simulink model "snap_f_12i_2kc"  (R2021a)
settings: Solver=VariableStepDiscrete  StartTime=0.0  StopTime=10.0  RelTol=1e-3
libraries: xbsIndex_r4 x2585, xps_library x8, casper_library_misc x8, casper_library_sources x4, casper_library_delays x2, casper_library_reorder x1, casper_library_communications x1
(part 1 of 32)
settings Model: ModifiedComment=kocz -- Fri Jun 12 15:44:21 2020 -- Version 1.371  Creator=mdexter  LastModifiedBy=jackh
settings Model: ModifiedHistory=|
  | kocz -- Fri Jun 12 15:36:18 2020 -- Version 1.370
  | 
  | Updated initial yellow blocks.
  | 
  | kocz -- Fri Jun 12 15:28:41 2020 -- Version 1.369
  | 
  | Started updating to 2018a. Restarting due to finding casper library bug.
  | 
  | jackh -- Sun Oct 27 09:17:26 2019 -- Version 1.368
  | compiled
  | 
  | jackh -- Sun Oct 27 07:24:12 2019 -- Version 1.367
  | remove registering of reorder outputs
  | 
  | jackh -- Sun Oct 27 07:22:37 2019 -- Version 1.366
  | change input snapshot to snap only one of 3 inputs
  | 
  | jackh -- Sun Oct 27 03:59:18 2019 -- Version 1.365
  | remove some superfluous registers to improve timing.
  | Reduce snapshot in input block from 1k samples to 512
  | 
  | jackh -- Sun Oct 27 01:46:50 2019 -- Version 1.364
  | Fix FFT shift bitwidth bug
  | 
  | FFT core was expecting a 16-bit shift, but only a 12bit value was sliced from the control register
  | 
  | jackh -- Fri Aug 30 09:22:01 2019 -- Version 1.363
  | compiled
  | 
  | jackh -- Thu Aug 29 17:13:27 2019 -- Version 1.362
  | change delay shift reg to 3 bit addr
  | 
  | jackh -- Thu Aug 29 11:33:13 2019 -- Version 1.361
  | corr fixes
  | 
  | jackh -- Thu Aug 29 11:09:21 2019 -- Version 1.360
  | latency fix in eqtvg
  | 
  | jackh -- Thu Aug 29 10:02:04 2019 -- Version 1.359
  | compiled
  | 
  | jackh -- Wed Aug 28 15:31:00 2019 -- Version 1.358
  | bump to version 1.3
  | 
  | jackh -- Wed Aug 28 15:26:18 2019 -- Version 1.357
  | change quantization to saturate.
  | Change coefficients to 16_5 (was 16_6)
  | 
  | jackh -- Wed Aug 28 14:17:28 2019 -- Version 1.356
  | remove debugging snapshots hidden in corr vaccs
  | 
  | jackh -- Fri Aug 23 15:01:55 2019 -- Version 1.355
  | compiled
  | 
  | jackh -- Fri Aug 23 10:43:05 2019 -- Version 1.354
  | add snapshot in input block
  | 
  | jackh -- Thu Aug 22 17:13:50 2019 -- Version 1.353
  | fix to eqtvg ram depths
  | 
  | jackh -- Thu Aug 22 15:23:14 2019 -- Version 1.352
  | bump version to 1.2
  | 
  | jackh -- Thu Aug 22 15:22:39 2019 -- Version 1.351
  | Force pairs of pols to have same random number generator to save resources
  | 
  | jackh -- Thu Aug 22 15:19:21 2019 -- Version 1.350
  | rotator channel index counter fixes
  | 
  | eq tvg split bram into 3 (so we can have 6 channels, not 8)
  | 
  | jackh -- Thu Aug 22 12:01:44 2019 -- Version 1.349
  | 
  | 
  | jackh -- Thu Aug 22 12:01:21 2019 -- Version 1.348
  | Changes to rotator precision
  | 
  | jackh -- Tue Aug 20 19:46:09 2019 -- Version 1.347
  | compiled
  | 
  | jackh -- Tue Aug 20 16:55:38 2019 -- Version 1.346
  | increase minimum walsh period to 2**18 fpga clocks (was 2**13)
  | 
  | jackh -- Tue Aug 20 16:40:34 2019 -- Version 1.345
  | 
  | 
  | jackh -- Tue Aug 20 16:15:18 2019 -- Version 1.344
  | bump version to 1.1
  | 
  | jackh -- Tue Aug 20 16:14:49 2019 -- Version 1.343
  | add global enables to phase switch mod/demod to make software easier
  | 
  | jackh -- Mon Aug 19 17:54:23 2019 -- Version 1.342
  | compiled
  | 
  | jackh -- Thu Aug 01 11:53:22 2019 -- Version 1.341
  | make programmable sync delay tolerate delay=0
  | 
  | jackh -- Wed Jul 31 13:49:54 2019 -- Version 1.340
  | comment out corr->rms
  | 
  | jackh -- Mon Jul 29 17:05:34 2019 -- Version 1.339
  | delete corr rms block (not currently enough ram)
  | 
  | jackh -- Mon Jul 29 17:03:29 2019 -- Version 1.338
  | Add version block
  | 
  | jackh -- Mon Jul 29 16:58:22 2019 -- Version 1.337
  | make sync in have a programmable delay
  | Solves 2 problems:
  | 
  | 1) Can start integrations at arbitrary times (good for LST alignment)
  | 2) Can start a 16 second integration chunk on an arbitrary time boundary (needed to avoid the downstream correlator having 16 second start / stop granularity)
  | 
  | jackh -- Mon Jul 29 16:50:03 2019 -- Version 1.336
  | update phasor to 24-bits
  | 
  | jackh -- Sat May 11 17:48:41 2019 -- Version 1.335
  | 
  | 
  | jackh -- Sat May 11 17:46:07 2019 -- Version 1.334
  | 
  | 
  | jackh -- Sat May 11 17:45:44 2019 -- Version 1.333
  | 
  | 
  | jackh -- Sat May 11 17:40:04 2019 -- Version 1.332
  | 
  | 
  | jackh -- Sat May 11 17:36:59 2019 -- Version 1.331
  | add vacc for autocorrs @ 16 bit resolution
  | 
  | deepthi -- Sun Oct 28 15:16:19 2018 -- Version 1.330
  | 
  | 
  | deepthi -- Sat Oct 27 18:45:54 2018 -- Version 1.329
  | 
  | packetizer: Added an 'and' block that holds new_packet signal in high until the first sync.
  | 
  | deepthi -- Sat Oct 27 17:33:32 2018 -- Version 1.328
  | 
  | 1. Change edge_detect location in sync block
  | 
  | deepthi -- Sat Oct 20 22:13:43 2018 -- Version 1.327
  | 
  | 1. Add edge detect to software reg and gpio input in sync block.
  | 
  | 2. Add new corr block with max hold functionality.
  | 
  | jackh -- Tue Oct 09 20:34:13 2018 -- Version 1.326
  | recompile with pmbus_alert register
  | 
  | jackh -- Thu Jul 12 10:55:28 2018 -- Version 1.325
  | 
  | 
  | jackh -- Wed Jul 11 17:20:51 2018 -- Version 1.324
  | syntax
  | 
  | jackh -- Wed Jul 11 17:16:24 2018 -- Version 1.323
  | increase resolution of phase rotator bram.
  | 
  | jackh -- Wed Jul 11 17:10:41 2018 -- Version 1.322
  | 
  | 
  | jackh -- Tue Jul 10 16:08:30 2018 -- Version 1.321
  | scramble rotator channel multiplers to match PFB output order (hopefully)
  | 
  | jackh -- Tue Jul 10 15:51:56 2018 -- Version 1.320
  | 
  | 
  | jackh -- Tue Jul 10 13:37:24 2018 -- Version 1.319
  | fix off-by-one in slicing of mcnt counter, which was having the effect of duplicating mcnts in headers
  | 
  | jackh -- Sat Jul 07 14:17:05 2018 -- Version 1.318
  | compiled
  | 
  | jackh -- Fri Jul 06 10:33:47 2018 -- Version 1.317
  | fix bitbashing to rotator phase addresses
  | 
  | jackh -- Fri Jul 06 10:17:15 2018 -- Version 1.316
  | Add mux to enable / disable rotator
  | 
  | jackh -- Thu Jul 05 17:21:10 2018 -- Version 1.315
  | make some delays behavioural
  | 
  | jackh -- Thu Jul 05 14:48:28 2018 -- Version 1.314
  | 
  | 
  | jackh -- Thu Jul 05 14:46:13 2018 -- Version 1.313
  | 
  | 
  | jackh -- Thu Jul 05 14:43:36 2018 -- Version 1.312
  | 
  | 
  | jackh -- Thu Jul 05 14:40:00 2018 -- Version 1.311
  | 
  | 
  | jackh -- Thu Jul 05 14:36:19 2018 -- Version 1.310
  | 
  | 
  | jackh -- Thu Jul 05 14:26:16 2018 -- Version 1.309
  | integrate rotator into pipeline
  | 
  | jackh -- Thu Jul 05 14:20:20 2018 -- Version 1.308
  | 
  | create phase-rotation block
  | 
  | deepthi -- Thu Jun 07 09:24:03 2018 -- Version 1.307
  | 
  | Replaced the corr block.
  | 
  | deepthi -- Wed Jun 06 12:07:26 2018 -- Version 1.306
  | 
  | 
  | deepthi -- Tue Jun 05 17:46:17 2018 -- Version 1.305
  | 
  | Replaced the corr block with the tested version
  | 
  | deepthi -- Sat May 12 19:11:02 2018 -- Version 1.304
  | 
  | Changed time counter to increment between even/odd banks
  | 
  | deepthi -- Sat May 12 19:06:34 2018 -- Version 1.303
  | 
  | changed timing of eof, valid, data and headers
  | 
  | deepthi -- Mon May 07 23:03:07 2018 -- Version 1.302
  | 
  | 
  | deepthi -- Mon May 07 00:31:44 2018 -- Version 1.301
  | 
  | 
  | deepthi -- Fri May 04 20:13:43 2018 -- Version 1.300
  | 
  | Reduced width sliced from time_ctr
  | 
  | deepthi -- Fri May 04 19:47:57 2018 -- Version 1.299
  | 
  | Added delay to header and ip signals to account for pulse_ext on valid.
  | 
  | deepthi -- Fri May 04 19:23:23 2018 -- Version 1.298
  | 
  | 
  | deepthi -- Thu May 03 16:58:39 2018 -- Version 1.297
  | 
  | 1. Added delays to eof and dest_ip  to account for pulse_ext in valid.
  | 
  | 2. Changed eth_sw expected packet length to include header.
  | 
  | jackh -- Tue May 01 20:38:09 2018 -- Version 1.296
  | compiled
  | 
  | jackh -- Tue May 01 17:49:38 2018 -- Version 1.295
  | Fix to packetizer valid generation, to take into account the 3 (one per antenna) blocks of valid data in each stream of 512 channels
  | 
  | jackh -- Tue May 01 16:49:02 2018 -- Version 1.294
  | make channel selection bram 32-bits wide.
  | 
  | Remove GPU-packing mux / swreg
  | 
  | jackh -- Tue May 01 14:24:16 2018 -- Version 1.293
  | 
  | 
  | jackh -- Tue May 01 14:20:01 2018 -- Version 1.292
  | update chan reorderer
  | 
  | jackh -- Tue May 01 11:43:41 2018 -- Version 1.291
  | compiled
  | 
  | jackh -- Tue May 01 09:44:03 2018 -- Version 1.290
  | 
  | 
  | jackh -- Tue May 01 09:43:34 2018 -- Version 1.289
  | use bram for eq fft descramble map
  | 
  | jackh -- Tue May 01 09:40:26 2018 -- Version 1.288
  | change architecture of corr block -- now stores desired antennas in bram, rather than using a delay tree
  | 
  | jackh -- Mon Apr 30 20:21:35 2018 -- Version 1.287
  | 
  | 
  | jackh -- Mon Apr 30 20:18:20 2018 -- Version 1.286
  | 
  | 
  | jackh -- Mon Apr 30 20:15:51 2018 -- Version 1.285
  | compensate for FFT scrambling in EQ block. Descramble FFT post-requantization in this block
  | 
  | jackh -- Mon Apr 30 19:27:42 2018 -- Version 1.284
  | plausibility pass on corr block
  | 
  | jackh -- Mon Apr 30 12:16:47 2018 -- Version 1.283
  | 
  | 
  | jackh -- Mon Apr 30 12:14:25 2018 -- Version 1.282
  | store chan_reorder reorder map in bram
  | 
  | jackh -- Mon Apr 30 12:05:02 2018 -- Version 1.281
  | remove per-antenna histograms -- now get one histogram with multiplexed input
  | 
  | jackh -- Sun Apr 29 15:50:16 2018 -- Version 1.280
  | 
  | 
  | jackh -- Sun Apr 29 15:37:38 2018 -- Version 1.279
  | 
  | 
  | jackh -- Sun Apr 29 15:27:38 2018 -- Version 1.278
  | First pass packetizer. Regenerate pfb with parameter for serial block inputs
  | 
  | jackh -- Sat Mar 03 12:52:57 2018 -- Version 1.277
  | 
  | 
  | jackh -- Sun Feb 25 12:27:48 2018 -- Version 1.276
  | add pre-pfb reorder
  | 
  | jackh -- Sat Feb 24 13:39:06 2018 -- Version 1.275
  | 
  | jackh -- Sat Feb 24 13:38:40 2018 -- Version 1.274
  | update pfb to 16 inputs
  | 
  | jackh -- Fri Feb 23 18:44:26 2018 -- Version 1.273
  | 
  | 
  | jackh -- Fri Feb 23 18:38:20 2018 -- Version 1.272
  | 
  | 
  | jackh -- Fri Feb 23 17:01:30 2018 -- Version 1.271
  | make fft 8 parallel input
  | 
  | jackh -- Sat Feb 10 13:53:12 2018 -- Version 1.270
  | 
  | 
  | jackh -- Sat Feb 10 13:50:10 2018 -- Version 1.269
  | 
  | 
  | jackh -- Sat Feb 10 13:48:56 2018 -- Version 1.268
  | remove fft preshift
  | 
  | jackh -- Sat Feb 10 13:47:39 2018 -- Version 1.267
  | 
  | 
  | jackh -- Sat Feb 10 13:44:29 2018 -- Version 1.266
  | 
  | 
  | jackh -- Sat Feb 10 13:43:22 2018 -- Version 1.265
  | make delayer dual-pol
  | 
  | jackh -- Sat Feb 10 13:40:59 2018 -- Version 1.264
  | first pass new packet format with no time-based corner turn
  | 
  | jackh -- Fri Feb 09 17:29:05 2018 -- Version 1.263
  | 
  | 
  | jackh -- Fri Feb 09 15:23:03 2018 -- Version 1.262
  | first pass turning everything to 8192 channels
  | 
  | Changed the ants addr to be driven by the same signal that drives chans, ips (used to be driven by ant_tracker).
  | 
  | Removed nants software register that was previously thought to control time stamps (but didn't really)
  | 
  | deepthi -- Wed Jan 31 18:20:45 2018 -- Version 1.261
  | 
  | deepthi -- Mon Jan 29 17:20:36 2018 -- Version 1.260
  | 
  | 
  | deepthi -- Mon Jan 29 17:18:54 2018 -- Version 1.259
  | 
  | 
  | deepthi -- Mon Jan 29 17:18:33 2018 -- Version 1.258
  | 
  | 
  | deepthi -- Mon Jan 29 16:51:19 2018 -- Version 1.257
  | 
  | 
  | deepthi -- Mon Jan 29 16:46:46 2018 -- Version 1.256
  | 
  | 
  | deepthi -- Mon Jan 29 16:37:32 2018 -- Version 1.255
  | 
  | 
  | deepthi -- Mon Jan 29 16:11:03 2018 -- Version 1.254
  | 
  | 
  | deepthi -- Mon Jan 29 15:55:33 2018 -- Version 1.253
  | 
  | 
  | jackh -- Fri Nov 17 19:04:05 2017 -- Version 1.252
  | compiled
  | 
  | jackh -- Wed Nov 15 11:31:03 2017 -- Version 1.251
  | go to 3 corr blocks
  | 
  | jackh -- Tue Nov 14 16:10:40 2017 -- Version 1.250
  | 
  | 
  | jackh -- Tue Nov 14 15:28:37 2017 -- Version 1.249
  | reduce bram use in histogram shared brams
  | 
  | jackh -- Mon Nov 13 18:55:18 2017 -- Version 1.248
  | fix bug in histogram shared bram addr width
  | 
  | jackh -- Fri Nov 10 17:05:56 2017 -- Version 1.247
  | add 4 independent corr subsystems. Add EQ clipping counters
  | 
  | jackh -- Fri Nov 10 14:21:14 2017 -- Version 1.246
  | 
  | 
  | jackh -- Fri Nov 10 14:19:27 2017 -- Version 1.245
  | 
  | 
  | jackh -- Fri Nov 10 11:40:47 2017 -- Version 1.244
  | update to histograms v2
  | 
  | jackh -- Tue Nov 07 22:23:59 2017 -- Version 1.243
  | compiled -- passes eqtvg
  | 
  | jackh -- Tue Nov 07 20:41:00 2017 -- Version 1.242
  | 
  | 
  | jackh -- Tue Nov 07 20:39:30 2017 -- Version 1.241
  | packet header generation fixes
  | 
  | jackh -- Tue Nov 07 17:19:53 2017 -- Version 1.240
  | 
  | 
  | jackh -- Tue Nov 07 17:14:47 2017 -- Version 1.239
  | 
  | 
  | jackh -- Tue Nov 07 17:08:29 2017 -- Version 1.238
  | remove some chan_reorder debug snapshots
  | 
  | jackh -- Tue Nov 07 17:06:39 2017 -- Version 1.237
  | update ps GPIO pins
  | 
  | **** Change packetizer header blocks to can have a separate antenna / ip / chan for each packet. This is for the nants > 3 simulation modes. This will break previous versions of software *****
  | 
  | jackh -- Mon Nov 06 22:06:03 2017 -- Version 1.236
  | add comment to corr_acc_len
  | 
  | Compiled -- passes EQTVG test!
  | 
  | jackh -- Mon Nov 06 15:24:31 2017 -- Version 1.235
  | add OR block in mrst generator so that counter is enabled if/when an arm signal comes
  | 
  | jackh -- Sun Nov 05 21:39:25 2017 -- Version 1.234
  | comment on sync period
  | 
  | jackh -- Sun Nov 05 17:39:01 2017 -- Version 1.233
  | fix bitbasher in 32-spectra corner turn
  | 
  | jackh -- Sun Nov 05 17:05:17 2017 -- Version 1.232
  | aesthetic
  | 
  | jackh -- Sun Nov 05 17:02:53 2017 -- Version 1.231
  | changes to comments
  | 
  | jackh -- Sun Nov 05 17:01:27 2017 -- Version 1.230
  | make acc_len it's own register so we can acc to 2**32
  | 
  | jackh -- Sun Nov 05 16:58:57 2017 -- Version 1.229
  | 
  | 
  | jackh -- Sun Nov 05 16:56:52 2017 -- Version 1.228
  | add internal correlator
  | 
  | jackh -- Sun Nov 05 16:24:21 2017 -- Version 1.227
  | compiled.
  | 
  | jackh -- Sun Nov 05 15:19:13 2017 -- Version 1.226
  | latency tweak to data line in packetizer
  | 
  | jackh -- Sat Nov 04 20:21:54 2017 -- Version 1.225
  | change ethernet debug counters to 32 bits
  | 
  | jackh -- Sat Nov 04 20:05:10 2017 -- Version 1.224
  | make chan reorder map bram 32 bits to aid with software
  | 
  | jackh -- Sat Nov 04 19:51:25 2017 -- Version 1.223
  | change header brams to be 32-bit wide for all values.
  | This makes it easier to deal with the software, which can only write 32-bit bounded words.
  | 
  | jackh -- Sat Nov 04 14:23:39 2017 -- Version 1.222
  | replace big distributed ram in 16-spectra corner turn
  | with simple bit basher manipulation. The distributed ram tool a ridiculous amount of time to synthesize. Hopefully this will be faster.
  | 
  | jackh -- Fri Nov 03 16:25:40 2017 -- Version 1.221
  | 
  | 
  | jackh -- Fri Nov 03 16:17:13 2017 -- Version 1.220
  | update casper blocks on phase switch subsys
  | 
  | jackh -- Fri Nov 03 16:14:34 2017 -- Version 1.219
  | 
  | 
  | jackh -- Fri Nov 03 13:09:23 2017 -- Version 1.218
  | add phase switching and i2c control
  | 
  | jackh -- Fri Nov 03 12:43:29 2017 -- Version 1.217
  | 
  | add i2C controllers
  | 
  | jackh -- Mon Oct 23 16:15:14 2017 -- Version 1.216
  | Add back in Deepthi's fix from f3b63dae07d62
  | 
  | jackh -- Mon Oct 23 16:04:59 2017 -- Version 1.215
  | 
  | 
  | jackh -- Mon Oct 23 14:44:02 2017 -- Version 1.214
  | compiled. Still minor timing errors in the histograms
  | 
  | jackh -- Mon Oct 23 10:40:37 2017 -- Version 1.213
  | change EQ coeffs to one-per channel. Make format 16_6 (was 18_7)
  | 
  | jackh -- Mon Oct 09 15:00:17 2017 -- Version 1.212
  | 
  | halve number of brams in histogram readout
  | 
  | jackh -- Wed Sep 13 11:46:17 2017 -- Version 1.211
  | use built-in tge status regs
  | 
  | jackh -- Tue Sep 12 21:14:25 2017 -- Version 1.210
  | 
  | 
  | jackh -- Tue Sep 12 21:10:57 2017 -- Version 1.209
  | update_casper_blocks(bdroot)
  | 
  | jackh -- Tue Sep 12 21:02:11 2017 -- Version 1.208
  | add histogram to adc stats
  | 
  | jackh -- Fri Jul 14 11:30:38 2017 -- Version 1.207
  | set map = reord_map in chan_reorder blocks which use matlab scripts to generate their reorders.
  | 
  | jackh -- Thu Jul 13 17:48:05 2017 -- Version 1.206
  | change sync period to a 32-bit sw reg (was hardcoded 9! * 1024)
  | 
  | deepthi -- Thu Jul 13 13:07:36 2017 -- Version 1.205
  | 
  | 
  | deepthi -- Thu Jul 13 12:10:35 2017 -- Version 1.204
  | 
  | 
  | deepthi -- Wed Jul 12 16:52:46 2017 -- Version 1.203
  | 
  | 
  | deepthi -- Wed Jul 12 15:57:48 2017 -- Version 1.202
  | 
  | 
  | deepthi -- Tue Jul 11 19:00:41 2017 -- Version 1.201
  | 
  | 
  | deepthi -- Tue Jul 11 18:54:05 2017 -- Version 1.200
  | 
  | 
  | deepthi -- Tue Jul 11 18:52:32 2017 -- Version 1.199
  | 
  | 
  | deepthi -- Mon Jul 10 16:18:51 2017 -- Version 1.198
  | 
  | 
  | deepthi -- Sun Jul 09 18:15:02 2017 -- Version 1.197
  | 
  | 
  | deepthi -- Thu Jul 06 13:54:16 2017 -- Version 1.196
  | 
  | 
  | jackh -- Mon Jul 03 11:01:40 2017 -- Version 1.195
  | 
  | 
  | jackh -- Fri Jun 30 13:59:17 2017 -- Version 1.194
  | enable CPU tx/rx buffer on tge core. Needed for microblaze.
  | 
  | jackh -- Mon Jun 26 11:33:24 2017 -- Version 1.193
  | 
  | 
  | jackh -- Thu Jun 22 14:37:16 2017 -- Version 1.192
  | add history prompting
settings SolverCC: AlgebraicLoopSolver=TrustRegion
settings DataIOCC: LimitDataPoints=on  SaveFormat=Array  SignalLoggingSaveFormat=ModelDataLogs  ReturnWorkspaceOutputs=off
settings OptimizationCC: DefaultParameterBehavior=Inlined  ExpressionDepthLimit=2147483647  LifeSpan=inf
settings DebuggingCC: UnderspecifiedInitializationDetection=Classic  MergeDetectMultiDrivingBlocksExec=none  SolverPrmCheckMsg=warning  FcnCallInpInsideContextMsg=warning  AllowSymbolicDim=off  StateNameClashWarn=warning  SFUnexpectedBacktrackingDiag=warning  SFNoUnconditionalDefaultTransitionDiag=warning  SFExecutionAtInitializationDiag=none  SFMachineParentedDataDiag=warning  ArithmeticOperatorsInVariantConditions=warning
settings HardwareCC: ProdBitPerPointer=32  ProdBitPerSizeT=32  ProdBitPerPtrDiffT=32  ProdLargestAtomicFloat=None  ProdIntDivRoundTo=Undefined  ProdEndianess=Unspecified  ProdWordSize=32  ProdHWDeviceType=32-bit Generic
settings ModelReferenceCC: PropagateSignalLabelsOutOfModel=off
settings SFSimCC: SimUseLocalCustomCode=off  CustomCodeUndefinedFunction=UseInterfaceOnly
settings RTWCC: RTWUseLocalCustomCode=off
settings CodeAppCC: StateflowObjectComments=on
settings GRTTargetCC: TargetLangStandard=C89/C90 (ANSI)  CombineOutputUpdateFcns=off  GRTInterface=on
settings ConfigComp: CovMetricSettings=dw  CovSaveCumulativeToWorkspaceVar=on  CovSaveSingleToWorkspaceVar=on  CovExternalEMLEnable=off

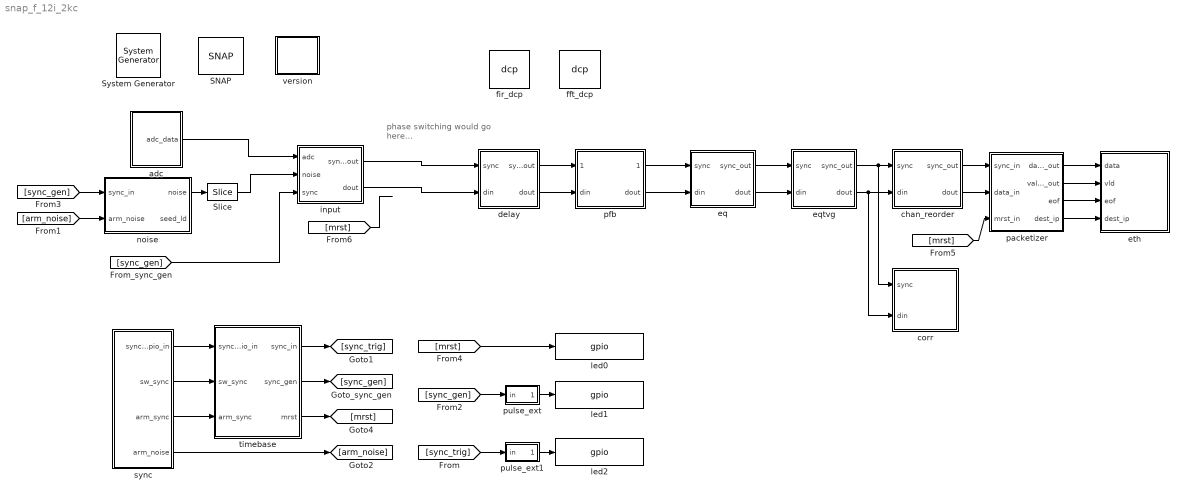
== system snap_f_12i_2kc ==
  note: phase switching
      | would go here...
  " System Generator" : xbsIndex_r4/ System Generator  Tag=genX  xilinxfamily=kintex7  part=xc7k160t  speed=-2  package=ffg676  synthesis_tool=XST  clock_wrapper=Clock Enables  directory=/home/jackh/src/cfa_snap_f/firmware/snap_f_12i_2kc/sysgen  proj_type=Vivado  Synth_file=Vivado Synthesis Defaults  Impl_file=Vivado Implementation Defaults  testbench=off  simulink_period=1  sysclk_period=4  dcm_input_clock_period=10  incr_netlist=off  trim_vbits=Everywhere in SubSystem  dbl_ovrd=According to Block Masks  core_generation=According to Block Masks  run_coregen=off  deprecated_control=off  eval_field=0  block_type=sysgen
  SNAP : xps_library/Platforms/SNAP  Tag=xps:xsg  hw_sys=SNAP:xc7k160t  clk_src=adc0_clk  clk_rate=250  use_microblaze=off  sample_period=1  synthesis_tool=XST
      settings: SourceProductName=CASPER XPS Blockset
  Slice : xbsIndex_r4/Slice  nbits=8*12  boolean_output=off  mode=Upper Bit Location + Width  bit1=0  base1=MSB of Input  bit0=0  base0=LSB of Input  dbl_ovrd=off  block_type=slice
  adc : Subsystem
  chan_reorder : Subsystem
  corr : Subsystem
  delay : Subsystem
  eq : Subsystem
  eqtvg : Subsystem
  eth : Subsystem
  fft_dcp : xps_library/Utilities/dcp  Tag=xps:dcp  dcp_file=[fileparts(which(gcs)) '/ip_cores/fft_12i_8192pt_18i18o_core/fft_12i_8192pt_18i18o_core.dcp']
      settings: SourceProductName=CASPER XPS Blockset
  fir_dcp : xps_library/Utilities/dcp  Tag=xps:dcp  dcp_file=[fileparts(which(gcs)) '/ip_cores/pfb_fir_12i_8192pt_8i18o_core/pfb_fir_12i_8192pt_8i18o_core.dcp']
      settings: SourceProductName=CASPER XPS Blockset
  input : Subsystem
  led0 : xps_library/IO/gpio  Tag=xps:gpio  io_group_params_forwarded=on  io_group=ROACH:led  io_group_real=led  io_group_custom=0  io_dir=out  arith_type=Boolean  bitwidth=1  bin_pt=0  bit_index=0  sample_period=1  use_single_ended=off  use_ddr=off  reg_iob=on  reg_clk_phase=0  termination=None  use_iodelay=off
      settings: SourceProductName=CASPER XPS Blockset
  led1 : xps_library/IO/gpio  Tag=xps:gpio  io_group_params_forwarded=on  io_group=ROACH:led  io_group_real=led  io_group_custom=0  io_dir=out  arith_type=Boolean  bitwidth=1  bin_pt=0  bit_index=1  sample_period=1  use_single_ended=off  use_ddr=off  reg_iob=on  reg_clk_phase=0  termination=None  use_iodelay=off
      settings: SourceProductName=CASPER XPS Blockset
  led2 : xps_library/IO/gpio  Tag=xps:gpio  io_group_params_forwarded=on  io_group=ROACH:led  io_group_real=led  io_group_custom=0  io_dir=out  arith_type=Boolean  bitwidth=1  bin_pt=0  bit_index=2  sample_period=1  use_single_ended=off  use_ddr=off  reg_iob=on  reg_clk_phase=0  termination=None  use_iodelay=off
      settings: SourceProductName=CASPER XPS Blockset
  noise : Subsystem
  packetizer : Subsystem  mask{nchan_bits=13, nsamp_per_pkt=2, nchan_per_pkt=384, nant_per_pkt=3, nants=4, clks_per_pkt=512/8*4*2*2, pkts_per_cycle=16*2, chan_frac_sent=384/512}
      mask prompts: nchan_bits "Number of channels (including unsent) (2^?)"; nsamp_per_pkt "Time samples per packet"; nchan_per_pkt "Channels per packet"; nant_per_pkt "Antennas per packet"; nants "Number of antennas including dummys"; clks_per_pkt "Send packet every ? clocks"; pkts_per_cycle "Packets per cycle"; chan_frac_sent "Fraction of channels sent"
      mask init:
      | nwords = nchan_per_pkt * nsamp_per_pkt * nant_per_pkt * 2 / 8
      | 
      | % +1 for dual-pol => 2 bytes per sample
      | % -3 for 2^3 = 8 bytes per word
      | 
      | clks_to_eof = (512*nsamp_per_pkt*nant_per_pkt*2/8) -(512*nsamp_per_pkt*2)/(4*8)
      | 
      | % 512 (including channels not sent)
      | % -512/4. to account for (1-chan_frac_sent) valid=0
  pfb : Subsystem
  pulse_ext : Subsystem  AncestorBlock=casper_library_misc/pulse_ext  mask(pulse_ext){pulse_len=2^26}
      mask prompts: pulse_len "Length of Pulse"
      mask help:
      | Extends a boolean signal to be high for the specified number of clocks after
      | the last high input.
      mask init:
      | bits = ceil(log2(pulse_len+1));
      mask Help: eval('xlWeb(''http://casper.berkeley.edu/wiki/Pulse_ext'')')
  pulse_ext1 : Subsystem  AncestorBlock=casper_library_misc/pulse_ext  mask(pulse_ext){pulse_len=2^26}
      mask prompts: pulse_len "Length of Pulse"
      mask help:
      | Extends a boolean signal to be high for the specified number of clocks after
      | the last high input.
      mask init:
      | bits = ceil(log2(pulse_len+1));
      mask Help: eval('xlWeb(''http://casper.berkeley.edu/wiki/Pulse_ext'')')
  sync : Subsystem
  timebase : Subsystem
  version : Subsystem  mask{ver_maj=1, ver_min=0}
      mask prompts: ver_maj "Major version"; ver_min "Minor version"
  wires:
  adc/1(adc_data) -> input/1(adc)
  noise/1(noise) -> Slice/1
  sync/1(sync_gpio_in) -> timebase/1(sync_gpio_in)
  sync/2(sw_sync) -> timebase/2(sw_sync)
  sync/3(arm_sync) -> timebase/3(arm_sync)
  [arm_noise] -> noise/2(arm_noise)
  [sync_gen] -> noise/1(sync_in)
  timebase/2(sync_gen) -> [sync_gen]
  timebase/1(sync_in) -> [sync_trig]
  sync/4(arm_noise) -> [arm_noise]
  [sync_gen] -> input/3(sync)
  eq/1(sync_out) -> eqtvg/1(sync)
  eq/2(dout) -> eqtvg/2(din)
  eqtvg/1(sync_out) -> corr/1(sync), chan_reorder/1(sync)
  eqtvg/2(dout) -> corr/2(din), chan_reorder/2(din)
  packetizer/1(data_out) -> eth/1(data)
  packetizer/2(valid_out) -> eth/2(vld)
  packetizer/3(eof) -> eth/3(eof)
  packetizer/4(dest_ip) -> eth/4(dest_ip)
  timebase/3(mrst) -> [mrst]
  [sync_gen] -> pulse_ext/1(in)
  [mrst] -> led0/1
  pulse_ext/1(out) -> led1/1
  delay/1(sync_out) -> pfb/1(sync_in)
  delay/2(dout) -> pfb/2(din)
  [sync_trig] -> pulse_ext1/1(in)
  pulse_ext1/1(out) -> led2/1
  input/2(dout) -> delay/2(din)
  input/1(sync_out) -> delay/1(sync)
  [mrst] -> ?
  chan_reorder/1(sync_out) -> packetizer/1(sync_in)
  chan_reorder/2(dout) -> packetizer/2(data_in)
  [mrst] -> packetizer/3(mrst_in)
  pfb/1(sync_out) -> eq/1(sync)
  pfb/2(dout) -> eq/2(din)
  Slice/1 -> input/2(noise)

== system snap_f_12i_2kc/adc ==
  Assert{,1..11} (12 alike) : xbsIndex_r4/Assert  assert_type=off  type_source=Explicitly  gui_display_data_type=Fixed-point  arith_type="Signed  (2's comp)"  n_bits=16  bin_pt=14  preci_type=Single  exp_width=8  frac_width=24  assert_rate=on  rate_source=Explicitly  period=1  output_port=on  block_type=assert
  Constant{4..13,33..34} (12 alike) : Constant  Value=0
  bus_create : Subsystem  AncestorBlock=casper_library_flow_control/bus_create  mask(bus_create){inputNum=12}
      mask prompts: inputNum "Number of inputs:"
      mask init:
      | bus_create_init(gcb,...
      |     'inputNum', inputNum);
  snap_adc : Subsystem  Tag=xps:snap_adc  AncestorBlock=xps_library/ADCs/snap_adc  mask(adc_snap){sample_rate=250, snap_inputs=12, adc_resolution=8}
      mask prompts: sample_rate "Sample rate (MHz)"; snap_inputs "Number of inputs per snap"; adc_resolution "Resolution of ADC (number of bit)"
      mask help: Interface to the 3 adc chips on the SNAP board. Please see Help for instructions on parameter settings
      mask init:
      | adc_snap_init(gcb);
      mask Help:
      | This is the CASPER "yellow block" for the ADCs on the SNAP board.
      | Each ADC chip accepts four inputs.
      | 
      | Maximum sample rate f (Mega samples per second)
      | 
      | Number of inputs         3                6                12
      | Resolution 8 bits          f=1000      f=500         f=250
      | Resolution 12 bits        f=640        f=320         f=160
      | 
      | Resolution 12 bits is available when SNAP board is upgraded with HMCAD1520 ADC chips
      mask TypeOptions snap_inputs: 3 | 6 | 12
      mask TypeOptions adc_resolution: 8 | 12
  adc_data : Outport  VectorParamsAs1DForOutWhenUnconnected=off
  wires:
  Constant4/1 -> snap_adc/1(a1_sim)
  Constant5/1 -> snap_adc/2(a2_sim)
  Constant6/1 -> snap_adc/3(a3_sim)
  Constant7/1 -> snap_adc/4(a4_sim)
  Constant8/1 -> snap_adc/5(b1_sim)
  Constant9/1 -> snap_adc/6(b2_sim)
  Constant33/1 -> snap_adc/7(b3_sim)
  Constant34/1 -> snap_adc/8(b4_sim)
  Constant10/1 -> snap_adc/9(c1_sim)
  Constant11/1 -> snap_adc/10(c2_sim)
  Constant12/1 -> snap_adc/11(c3_sim)
  Constant13/1 -> snap_adc/12(c4_sim)
  bus_create/1(bus_out) -> adc_data/1
  snap_adc/1(a1) -> Assert/1  "in0"
  snap_adc/2(a2) -> Assert1/1  "in1"
  snap_adc/3(a3) -> Assert2/1  "in2"
  snap_adc/4(a4) -> Assert3/1  "in3"
  snap_adc/5(b1) -> Assert4/1  "in4"
  snap_adc/6(b2) -> Assert5/1  "b2"
  snap_adc/7(b3) -> Assert6/1  "b3"
  snap_adc/8(b4) -> Assert7/1  "b4"
  snap_adc/9(c1) -> Assert8/1  "c1"
  snap_adc/10(c2) -> Assert9/1  "c2"
  snap_adc/11(c3) -> Assert10/1  "c3"
  snap_adc/12(c4) -> Assert11/1  "c4"
  Assert/1 -> bus_create/1(in1)
  Assert1/1 -> bus_create/2(in2)
  Assert2/1 -> bus_create/3(in3)
  Assert3/1 -> bus_create/4(in4)
  Assert6/1 -> bus_create/7(in7)
  Assert7/1 -> bus_create/8(in8)
  Assert5/1 -> bus_create/6(in6)
  Assert4/1 -> bus_create/5(in5)
  Assert9/1 -> bus_create/10(in10)
  Assert8/1 -> bus_create/9(in9)
  Assert11/1 -> bus_create/12(in12)
  Assert10/1 -> bus_create/11(in11)

== system snap_f_12i_2kc/chan_reorder ==
  note: insert zeros so order is now:
      |
      | 4096 chans x 2 ants x [4 ants x 2 pols]
      |
      | And antennas 3, 7, 11, 15 are zero
      |
      | Equivalent to:
      |
      | 2048 chans x 2 chans x 2 ants x [4 ants x 2 pols]
  note: remap serially so order is:
      |
      | 4096 chans x 2 inputs x [6 inputs]
      |
      | Let's call this:
      |
      | 4096 chans x 2 ants x [3 ants x 2 pols]
  note: input order is:
      | a0, a1, ..., a4095, b0, b1, ..., b4095
      | ...
      | k0, k1, ..., k4095, l0, l1, ..., l4095
      |
      | (i.e., 6 inputs in parallel, with two inputs in serial)
      | A complete cycle takes 2 x 4096 (channels) = 8192 clocks
  note: After square transpose:
      |
      | 2048 chans x 4 ants x [2 chans x 2 ants x 2 pols]
      |
      | And antennas 3, 7, 11, 15 are zero
  sync : Inport
  din : Inport  Port=2
  Constant2 : xbsIndex_r4/Constant  const=1  gui_display_data_type=Boolean  arith_type=Boolean  n_bits=1  bin_pt=0  preci_type=Single  exp_width=8  frac_width=24  explicit_period=on  period=1  equ=P=C  opselect=C  inp2=PCIN>>17  opr=+  inp1=P  carry=CIN  dbl_ovrd=off  block_type=constant
  Constant3 : xbsIndex_r4/Constant  const=0  gui_display_data_type=Fixed-point  arith_type=Unsigned  n_bits=16  bin_pt=0  preci_type=Single  exp_width=8  frac_width=24  explicit_period=on  period=1  equ=P=C  opselect=C  inp2=PCIN>>17  opr=+  inp1=P  carry=CIN  dbl_ovrd=off  block_type=constant
  bus_create : Subsystem  AncestorBlock=casper_library_flow_control/bus_create  mask(bus_create){inputNum=4}
      mask prompts: inputNum "Number of inputs:"
      mask init:
      | bus_create_init(gcb,...
      |     'inputNum', inputNum);
  bus_expand3 : Subsystem  AncestorBlock=casper_library_flow_control/bus_expand  mask(bus_expand){mode=divisions of equal size, outputNum=3, outputWidth=8*2, outputBinaryPt=0, outputArithmeticType=0, show_format=off, outputToWorkspace=off, variablePrefix=out, outputToModelAsWell=on}
      mask prompts: outputNum "Number of outputs:"; outputWidth "Output width:"; outputBinaryPt "Output binary point position:"; outputArithmeticType "Output arithmetic type (ufix=0, fix=1, bool=2):"; show_format "Print format string?"; outputToWorkspace "Output to workspace?"; variablePrefix "Variable name prefix:"; outputToModelAsWell "Output to model as well?"
      mask help:
      | Expands a 'bus' made using a bus_create or Xilinx
      | concat block.
      | The input will be divided into the specified number
      | of outputs with the specified arithmetic types.
      | Divisions are made from most significant bit.
      mask init:
      | bus_expand_init(gcb,...
      |     'mode', mode, ...
      |     'outputNum', outputNum, ...
      |     'outputWidth', outputWidth, ...
      |     'outputBinaryPt', outputBinaryPt, ...
      |     'outputArithmeticType', outputArithmeticType, ...
      |     'show_format', show_format, ...
      |     'outputToWorkspace', outputToWorkspace, ...
      |     'variablePrefix', variablePrefix, ...
      |     'outputToModelAsWell', outputToModelAsWell);
      settings: AttributesFormatString=3 outputs
      mask TypeOptions mode: divisions of equal size | divisions of arbitrary size
      mask Callback mode: %bus_expand_callback();
      mask Callback outputWidth: %bus_expand_callback();
      mask Callback outputToWorkspace: %bus_expand_callback();
  reorder3 : Subsystem  AncestorBlock=casper_library_reorder/reorder  mask(reorder){map=[0:8191], n_bits=0, n_inputs=1, bram_latency=3, map_latency=3, fanout_latency=0, double_buffer=1, bram_map=on, software_controlled=on, use_control_fanout=on, hide_latency=off}
      mask prompts: map "Output Order:"; n_bits "Data width in"; n_inputs "Number of inputs"; bram_latency "BRAM Latency"; map_latency "Map Latency"; fanout_latency "Fanout latency"; double_buffer "Double Buffer"; bram_map "Use BlockRAM for Map"; software_controlled "Use runtime software control"; use_control_fanout "Control fanout of control to multiple iniputs"; hide_latency "EXPERIMENTAL: Hide control latency"
      mask init:
      | reorder_init(gcb, ...
      |     'map', map, ...
      |     'n_bits', n_bits, ...
      |     'n_inputs', n_inputs, ...
      |     'bram_latency', bram_latency, ...
      |     'map_latency', map_latency, ...
      |     'fanout_latency', fanout_latency, ...
      |     'double_buffer', double_buffer, ...
      |     'bram_map', bram_map, ...
      |     'software_controlled', software_controlled, ...
      |     'use_control_fanout', use_control_fanout, ...
      |     'hide_latency', hide_latency);
      settings: AttributesFormatString=order=2
      mask Help: eval('xlWeb(''http://casper.berkeley.edu/wiki/Reorder'')')
  square_transposer3 : Subsystem  AncestorBlock=casper_library_reorder/square_transposer  mask(square_transposer){n_inputs=2, async=off}
      mask prompts: n_inputs "Number of inputs (2^?):"; async "Aynchronus operation"
      mask init:
      | square_transposer_init(gcb,...
      |     'n_inputs', n_inputs, ...
      |     'async', async);
      settings: AttributesFormatString=n_inputs=2
      mask Help: eval('xlWeb(''http://casper.berkeley.edu/wiki/Square_transposer'')')
  sync_out : Outport  VectorParamsAs1DForOutWhenUnconnected=off
  dout : Outport  Port=2  VectorParamsAs1DForOutWhenUnconnected=off
  wires:
  square_transposer3/1(sync_out) -> sync_out/1
  Constant2/1 -> reorder3/2(en)
  sync/1 -> reorder3/1(sync)
  din/1 -> reorder3/3(din0)
  reorder3/2(valid) -> ?
  reorder3/3(dout0) -> bus_expand3/1(bus_in)
  reorder3/1(sync_out) -> square_transposer3/1(sync)
  bus_expand3/1(msb_out3) -> square_transposer3/2(in0)
  bus_expand3/2(out2) -> square_transposer3/3(in1)
  bus_expand3/3(lsb_out1) -> square_transposer3/4(in2)
  Constant3/1 -> square_transposer3/5(in3)
  square_transposer3/3(out1) -> bus_create/2(in2)
  square_transposer3/4(out2) -> bus_create/3(in3)
  square_transposer3/2(out0) -> bus_create/1(in1)
  square_transposer3/5(out3) -> bus_create/4(in4)
  bus_create/1(bus_out) -> dout/1

== system snap_f_12i_2kc/corr ==
  sync : Inport
  din : Inport  Port=2
  0 : Subsystem  mask{nchan_bits=12, npol_bits=1}
      mask prompts: nchan_bits "Number of channels (2^?)"; npol_bits "Number of pols (2^?)"
  wires:
  sync/1 -> 0/1(sync)
  din/1 -> 0/2(din)

== system snap_f_12i_2kc/delay ==
  sync : Inport
  din : Inport  Port=2
  Delay1 : xbsIndex_r4/Delay  rst=off  infoeditControl=Selection of Reset will increase slice count due to use of real FFs and instead of SRLs  en=off  latency=1  reg_retiming=on  dbl_ovrd=off  block_type=delay
  delayer : Subsystem
  delays : Subsystem  Tag=xps:sw_reg  AncestorBlock=xps_library/Memory/software_register  mask(swreg){io_dir=From Processor, io_delay=0, init_val=0, sample_period=1, names=reg, bitwidths=32, bin_pts=0, arith_types=0, sim_port=on, show_format=off}
      mask prompts: io_dir "I/O direction"; io_delay "I/O delay"; init_val "Initial Value"; sample_period "Sample period"; names "Bitfield names [msb...lsb]"; bitwidths "Bitfield widths"; bin_pts "Bitfield binary pts"; arith_types "Bitfield types, ufix=0, fix=1, bool=2"; sim_port "Provide sim input/output?"; show_format "Print format string?"
      mask help: A 32-bit software-accessible register. Can be divided into bitfields of varying widths and types using the fields in the block mask.
      mask init:
      | swreg_init(gcb)
      settings: AttributesFormatString=1input
      mask TypeOptions io_dir: To Processor | From Processor
      mask Callback io_dir:
      | mask_enables = get_param(gcb, 'MaskEnables');
      | mask_names = get_param(gcb, 'MaskNames');
      | if strcmp(get_param(gcb, 'io_dir'), 'To Processor'),
      |     mask_enables{ismember(mask_names, 'sample_period')} = 'off';
      | else
      |     mask_enables{ismember(mask_names, 'sample_period')} = 'on';
      | end
      | set_param(gcb, 'MaskEnables', mask_enables);
      mask DialogControl ParameterTabVar0 Prompt: Setup
  sync_out : Outport  VectorParamsAs1DForOutWhenUnconnected=off
  dout : Outport  Port=2  VectorParamsAs1DForOutWhenUnconnected=off
  wires:
  delays/1(in_reg) -> delayer/1(delays)
  din/1 -> delayer/2(din)
  delayer/1(dout) -> dout/1
  sync/1 -> Delay1/1
  Delay1/1 -> sync_out/1

== system snap_f_12i_2kc/eq ==
  note: After quantizing, do the final stage of the FFT descramble.
      | With 4-, rather than 18-bit values, it'll use 25% of the BRAM.
  sync : Inport
  din : Inport  Port=2
  core : Subsystem  mask{nchan=12, nants=2}
      mask prompts: nchan "Number of fft channels (2^?)"; nants "Number of Antennas"
  sync_out : Outport  VectorParamsAs1DForOutWhenUnconnected=off
  dout : Outport  Port=2  VectorParamsAs1DForOutWhenUnconnected=off
  wires:
  din/1 -> core/2(in)
  sync/1 -> core/1(sync)
  core/2(dout) -> dout/1  "data"
  core/1(sync_out) -> sync_out/1

== system snap_f_12i_2kc/eqtvg ==
  sync : Inport
  din : Inport  Port=2
  Constant1 : xbsIndex_r4/Constant  const=0  gui_display_data_type=Fixed-point  arith_type=Unsigned  n_bits=16  bin_pt=0  preci_type=Single  exp_width=8  frac_width=24  explicit_period=on  period=1  equ=P=C  opselect=C  inp2=PCIN>>17  opr=+  inp1=P  carry=CIN  dbl_ovrd=off  block_type=constant
  Constant2 : xbsIndex_r4/Constant  const=0  gui_display_data_type=Fixed-point  arith_type=Unsigned  n_bits=16  bin_pt=0  preci_type=Single  exp_width=8  frac_width=24  explicit_period=on  period=1  equ=P=C  opselect=C  inp2=PCIN>>17  opr=+  inp1=P  carry=CIN  dbl_ovrd=off  block_type=constant
  Constant3 : xbsIndex_r4/Constant  const=0  gui_display_data_type=Boolean  arith_type=Boolean  n_bits=64  bin_pt=0  preci_type=Single  exp_width=8  frac_width=24  explicit_period=on  period=1  equ=P=C  opselect=C  inp2=PCIN>>17  opr=+  inp1=P  carry=CIN  dbl_ovrd=off  block_type=constant
  Constant4 : xbsIndex_r4/Constant  const=0  gui_display_data_type=Boolean  arith_type=Boolean  n_bits=64  bin_pt=0  preci_type=Single  exp_width=8  frac_width=24  explicit_period=on  period=1  equ=P=C  opselect=C  inp2=PCIN>>17  opr=+  inp1=P  carry=CIN  dbl_ovrd=off  block_type=constant
  Constant5 : xbsIndex_r4/Constant  const=0  gui_display_data_type=Fixed-point  arith_type=Unsigned  n_bits=16  bin_pt=0  preci_type=Single  exp_width=8  frac_width=24  explicit_period=on  period=1  equ=P=C  opselect=C  inp2=PCIN>>17  opr=+  inp1=P  carry=CIN  dbl_ovrd=off  block_type=constant
  Constant6 : xbsIndex_r4/Constant  const=0  gui_display_data_type=Boolean  arith_type=Boolean  n_bits=64  bin_pt=0  preci_type=Single  exp_width=8  frac_width=24  explicit_period=on  period=1  equ=P=C  opselect=C  inp2=PCIN>>17  opr=+  inp1=P  carry=CIN  dbl_ovrd=off  block_type=constant
  Counter : xbsIndex_r4/Counter  cnt_type=Count Limited  cnt_to=2^(12) * 2 - 1  operation=Up  start_count=0  cnt_by_val=1  arith_type=Unsigned  n_bits=ceil(log2(2^(12) * 2))  bin_pt=0  load_pin=off  rst=on  en=off  explicit_period=on  period=1  use_behavioral_HDL=off  implementation=Fabric  dbl_ovrd=off  block_type=counter
  Delay1 : xbsIndex_r4/Delay  rst=off  infoeditControl=Selection of Reset will increase slice count due to use of real FFs and instead of SRLs  en=off  latency=1  reg_retiming=off  dbl_ovrd=off  block_type=delay
  Delay2 : xbsIndex_r4/Delay  rst=off  infoeditControl=Selection of Reset will increase slice count due to use of real FFs and instead of SRLs  en=off  latency=3  reg_retiming=off  dbl_ovrd=off  block_type=delay
  Delay3 : xbsIndex_r4/Delay  rst=off  infoeditControl=Selection of Reset will increase slice count due to use of real FFs and instead of SRLs  en=off  latency=3  reg_retiming=on  dbl_ovrd=off  block_type=delay
  Delay4 : xbsIndex_r4/Delay  rst=off  infoeditControl=Selection of Reset will increase slice count due to use of real FFs and instead of SRLs  en=off  latency=3  reg_retiming=on  dbl_ovrd=off  block_type=delay
  Mux : xbsIndex_r4/Mux  inputs=2  en=off  latency=1  precision=Full  arith_type=Unsigned  n_bits=16  bin_pt=14  quantization=Truncate  overflow=Wrap  dbl_ovrd=off  block_type=mux
  Slice : xbsIndex_r4/Slice  nbits=1  boolean_output=on  mode=Lower Bit Location + Width  bit1=0  base1=MSB of Input  bit0=0  base0=LSB of Input  dbl_ovrd=off  block_type=slice
  bus_create : Subsystem  AncestorBlock=casper_library_flow_control/bus_create  mask(bus_create){inputNum=3}
      mask prompts: inputNum "Number of inputs:"
      mask init:
      | bus_create_init(gcb,...
      |     'inputNum', inputNum);
  tv0 : Subsystem  Tag=xps:bram  AncestorBlock=xps_library/Memory/shared_bram  mask{arith_type=Unsigned, addr_width=ceil(log2(2^(12)*2)), data_width=16, reg_prim_output=on, reg_core_output=on, optimization=Minimum_Area, data_bin_pt=0, init_vals=[0:2^13-1], sample_rate=1}
      mask prompts: arith_type "Output Data Type"; addr_width "Address width"; data_width "Data Width"; reg_prim_output "Register Primitive Output"; reg_core_output "Register Core Output"; data_bin_pt "Data Binary Point"; init_vals "Initial values (simulation only)"; sample_rate "Sample rate"
      mask init:
      | shared_bram_mask;
      mask TypeOptions arith_type: Unsigned | Signed  (2's comp)
      mask TypeOptions data_width: 8 | 16 | 32 | 64 | 128
      mask TypeOptions optimization: Minimum_Area | Low_Power
  tv1 : Subsystem  Tag=xps:bram  AncestorBlock=xps_library/Memory/shared_bram  mask{arith_type=Unsigned, addr_width=ceil(log2(2^(12)*2)), data_width=16, reg_prim_output=on, reg_core_output=on, optimization=Minimum_Area, data_bin_pt=0, init_vals=[0:2^13-1], sample_rate=1}
      mask prompts: arith_type "Output Data Type"; addr_width "Address width"; data_width "Data Width"; reg_prim_output "Register Primitive Output"; reg_core_output "Register Core Output"; data_bin_pt "Data Binary Point"; init_vals "Initial values (simulation only)"; sample_rate "Sample rate"
      mask init:
      | shared_bram_mask;
      mask TypeOptions arith_type: Unsigned | Signed  (2's comp)
      mask TypeOptions data_width: 8 | 16 | 32 | 64 | 128
      mask TypeOptions optimization: Minimum_Area | Low_Power
  tv2 : Subsystem  Tag=xps:bram  AncestorBlock=xps_library/Memory/shared_bram  mask{arith_type=Unsigned, addr_width=ceil(log2(2^(12)*2)), data_width=16, reg_prim_output=on, reg_core_output=on, optimization=Minimum_Area, data_bin_pt=0, init_vals=[0:2^13-1], sample_rate=1}
      mask prompts: arith_type "Output Data Type"; addr_width "Address width"; data_width "Data Width"; reg_prim_output "Register Primitive Output"; reg_core_output "Register Core Output"; data_bin_pt "Data Binary Point"; init_vals "Initial values (simulation only)"; sample_rate "Sample rate"
      mask init:
      | shared_bram_mask;
      mask TypeOptions arith_type: Unsigned | Signed  (2's comp)
      mask TypeOptions data_width: 8 | 16 | 32 | 64 | 128
      mask TypeOptions optimization: Minimum_Area | Low_Power
  tvg_en : Subsystem  Tag=xps:sw_reg  AncestorBlock=xps_library/Memory/software_register  mask(swreg){io_dir=From Processor, io_delay=0, init_val=0, sample_period=1, names=reg, bitwidths=32, bin_pts=0, arith_types=0, sim_port=on, show_format=off}
      mask prompts: io_dir "I/O direction"; io_delay "I/O delay"; init_val "Initial Value"; sample_period "Sample period"; names "Bitfield names [msb...lsb]"; bitwidths "Bitfield widths"; bin_pts "Bitfield binary pts"; arith_types "Bitfield types, ufix=0, fix=1, bool=2"; sim_port "Provide sim input/output?"; show_format "Print format string?"
      mask help: A 32-bit software-accessible register. Can be divided into bitfields of varying widths and types using the fields in the block mask.
      mask init:
      | swreg_init(gcb)
      settings: AttributesFormatString=1input
      mask TypeOptions io_dir: To Processor | From Processor
      mask Callback io_dir:
      | mask_enables = get_param(gcb, 'MaskEnables');
      | mask_names = get_param(gcb, 'MaskNames');
      | if strcmp(get_param(gcb, 'io_dir'), 'To Processor'),
      |     mask_enables{ismember(mask_names, 'sample_period')} = 'off';
      | else
      |     mask_enables{ismember(mask_names, 'sample_period')} = 'on';
      | end
      | set_param(gcb, 'MaskEnables', mask_enables);
      mask DialogControl ParameterTabVar0 Prompt: Setup
  sync_out : Outport  VectorParamsAs1DForOutWhenUnconnected=off
  dout : Outport  Port=2  VectorParamsAs1DForOutWhenUnconnected=off
  wires:
  din/1 -> Delay3/1
  Delay1/1 -> sync_out/1  "sync"
  tvg_en/1(in_reg) -> Slice/1
  sync/1 -> Delay2/1, Counter/1
  Mux/1 -> dout/1
  Slice/1 -> Delay4/1
  Constant2/1 -> tv0/2(data_in)
  Constant3/1 -> tv0/3(we)
  Delay4/1 -> Mux/1
  Delay3/1 -> Mux/2
  bus_create/1(bus_out) -> Mux/3
  Constant1/1 -> tv1/2(data_in)
  Constant4/1 -> tv1/3(we)
  Constant5/1 -> tv2/2(data_in)
  Constant6/1 -> tv2/3(we)
  Delay2/1 -> Delay1/1
  Counter/1 -> tv2/1(addr), tv1/1(addr), tv0/1(addr)
  tv2/1(data_out) -> bus_create/3(in3)
  tv1/1(data_out) -> bus_create/2(in2)
  tv0/1(data_out) -> bus_create/1(in1)
